simulink model "RTS_15km"  (R2018a)
settings: Solver=ode15s  StartTime=0.0  StopTime=20  FixedStep=0.00001  RelTol=1e-3  AbsTol=1e-6
values from neighbouring files (symbols this model uses):
  ADAMS_cwd = 'C:\Users\gct14001\Documents\Latest DECEMBER Bike Model\Simulation Files'    [Nonlinear_Torque_15km.m]
  ADAMS_exec = ''    [Nonlinear_Torque_15km.m]
  ADAMS_host = 'DESKTOP-F3FKN9V.mdh.se'    [Nonlinear_Torque_15km.m]
  ADAMS_init = ''    [Nonlinear_Torque_15km.m]
  ADAMS_inputs = 'TorqueMotor.var_motor_torque!V_In!FrameDisturbance'    [Nonlinear_Torque_15km.m]
  ADAMS_outputs = 'LeanAng_In!SteerAngle!V_Out!Dist!DriftAngle'    [Nonlinear_Torque_15km.m]
  ADAMS_prefix = 'Nonlinear_Torque_15km'    [Nonlinear_Torque_15km.m]
  ADAMS_static = 'no'    [Nonlinear_Torque_15km.m]
  ADAMS_sysdir = 'C:\PROGRA~1\MSC~1.SOF\ADAMSS~1\2018_1\'    [Nonlinear_Torque_15km.m]
  Cline = v*inv(M)*C1    [DynamicModelParameters.m]
  Kline = inv(M)*(g*K0+v^2*K2)    [DynamicModelParameters.m]
  Mline = inv(M)    [DynamicModelParameters.m]
libraries: simulink_extras x3, simulink x2, dspfdesign x1
settings Model: Creator=FoR  LastModifiedBy=gct14001
settings SolverCC: SolverResetMethod=Robust
settings CodeAppCC: StateflowObjectComments=on

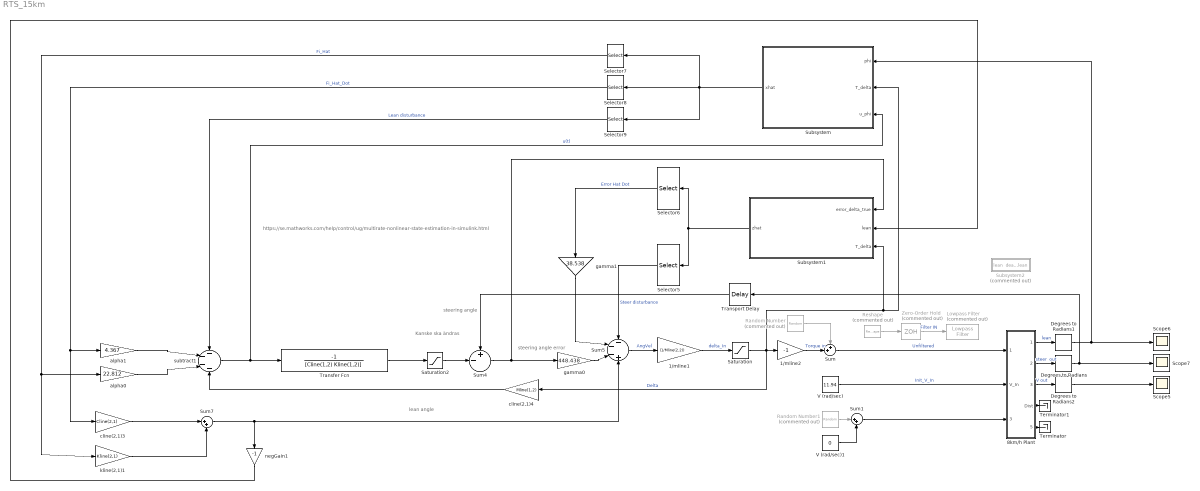
== system RTS_15km ==
  note: steering angle
  note: https://se.mathworks.com/help/control/ug/multirate-nonlinear-state-estimation-in-simulink.html
  note: steering angle error
  note: Kanske ska
      | ändras
  note: lean angle
  1/mline1 : Gain  Gain=(1/Mline(2,2))
  1/mline2 : Gain  Gain=-1
  8km/h Plant : Subsystem
  Degrees to Radians : simulink_extras/Transformations/Degrees to Radians
  Degrees to Radians1 : simulink_extras/Transformations/Degrees to Radians
  Degrees to Radians2 : simulink_extras/Transformations/Degrees to Radians
  Lowpass Filter : dspfdesign/Lowpass Filter  Commented=on  FilterType=FIR  DesignForMinimumOrder=on  FilterOrder=50  PassbandFrequency=15  StopbandFrequency=50  PassbandRipple=0.1  StopbandAttenuation=80  InheritSampleRate=off  SampleRate=44100  SimulateUsing=Interpreted execution  roundingMode=Floor  coeffsDataTypeStr=fixdt(1,16)
  Random Number : RandomNumber  Commented=on  Variance=0.1  SampleTime=0.1
  Random Number1 : RandomNumber  Commented=on  Variance=0.1  SampleTime=0.1
  Reshape : Reshape  Commented=on  OutputDimensionality=Customize  OutputDimensions=1
  Saturation : Saturate  UpperLimit=12  LowerLimit=-12
  Saturation2 : Saturate  UpperLimit=90  LowerLimit=-90
  Scope5 : Scope
  Scope6 : Scope
  Scope7 : Scope
  Selector5 : Selector  InputPortWidth=6  IndexOptions=Index vector (dialog)  Indices=3  OutputSizes=1
  Selector6 : Selector  InputPortWidth=6  IndexOptions=Index vector (dialog)  Indices=2  OutputSizes=1
  Selector7 : Selector  InputPortWidth=3  IndexOptions=Index vector (dialog)  Indices=1  OutputSizes=1
  Selector8 : Selector  InputPortWidth=3  IndexOptions=Index vector (dialog)  Indices=2  OutputSizes=1
  Selector9 : Selector  InputPortWidth=3  IndexOptions=Index vector (dialog)  Indices=3  OutputSizes=1
  Subsystem : Subsystem
  Subsystem1 : Subsystem
  Subsystem2 : Subsystem  Commented=on
  Sum : Sum  Inputs=++|
  Sum1 : Sum  Inputs=|++
  Sum4 : Sum  Inputs=+-|
  Sum5 : Sum  Inputs=---+
  Sum7 : Sum  Inputs=|++
  Terminator : Terminator
  Terminator1 : Terminator
  Transfer Fcn : TransferFcn  Numerator=[-1]  Denominator=[Cline(1,2) Kline(1,2)]
  Transport Delay : TransportDelay  DelayTime=0.005
  V (rad/sec) : Constant  Value=11.94
  V (rad/sec)1 : Constant  Value=0
  Zero-Order Hold : ZeroOrderHold  Commented=on  SampleTime=-1
  alpha0 : Gain  Gain=22.812
  alpha1 : Gain  Gain=4.367
  cline(2,1)3 : Gain  Gain=Cline(2,1)
  cline(2,1)4 : Gain  Gain=Mline(1,2)
  gamma0 : Gain  Gain=448.438
  "gamma1 " : Gain  Gain=38.538
  kline(2,1)1 : Gain  Gain=Kline(2,1)
  negGain1 : Gain  Gain=-1
  subtract1 : Sum  Inputs=----
  wires:
  Saturation/1 -> 1/mline2/1, cline(2,1)4/1, Subsystem1/3(T_delta), Subsystem/2(T_delta)  "Delta"
  Subsystem1/1(zhat) -> Selector5/1, Selector6/1
  Selector7/1 -> kline(2,1)1/1, alpha0/1  "Fi_Hat"
  cline(2,1)3/1 -> Sum7/1
  Selector9/1 -> subtract1/1  "Lean disturbance"
  cline(2,1)4/1 -> subtract1/4
  Selector5/1 -> Sum5/1  "Steer disturbance"
  Sum7/1 -> negGain1/1, Sum5/4
  Sum5/1 -> 1/mline1/1  "AngVel"
  alpha0/1 -> subtract1/3
  alpha1/1 -> subtract1/2
  gamma0/1 -> Sum5/3
  kline(2,1)1/1 -> Sum7/2
  subtract1/1 -> Transfer Fcn/1, Subsystem/3(u_phi)  "u(t)"
  1/mline1/1 -> Saturation/1  "delta_In"
  Selector8/1 -> cline(2,1)3/1, alpha1/1  "Fi_Hat_Dot"
  8km/h Plant/3("V_Out     ") -> Degrees to Radians2/1  "V out"
  "gamma1 "/1 -> Sum5/2
  Sum4/1 -> Subsystem1/1(error_delta_true), gamma0/1
  Selector6/1 -> "gamma1 "/1  "Error Hat Dot"
  Saturation2/1 -> Sum4/2
  negGain1/1 -> Subsystem1/2(lean)
  Subsystem/1(xhat) -> Selector9/1, Selector8/1, Selector7/1
  V (rad/sec)/1 -> 8km/h Plant/2("V_In                        ")  "Init_V_In"
  8km/h Plant/4("Dist      ") -> Terminator1/1
  8km/h Plant/5(DriftAngle) -> Terminator/1
  8km/h Plant/2(SteerAngle) -> Degrees to Radians/1  "steer  out"
  Transfer Fcn/1 -> Saturation2/1
  Degrees to Radians/1 -> Scope7/1, Transport Delay/1
  Transport Delay/1 -> Sum4/1
  Degrees to Radians1/1 -> Subsystem/1(phi), Scope6/1
  1/mline2/1 -> Sum/2  "Torque in"
  Random Number/1 -> Sum/1
  8km/h Plant/1(LeanAng_In) -> Degrees to Radians1/1  "lean"
  V (rad/sec)1/1 -> Sum1/2
  Degrees to Radians2/1 -> Scope5/1
  Random Number1/1 -> Sum1/1
  Sum1/1 -> 8km/h Plant/3("FrameDisturbance            ")
  Sum/1 -> 8km/h Plant/1(TorqueMotor.var_motor_torque)  "Unfiltered"
  Reshape/1 -> Zero-Order Hold/1
  Zero-Order Hold/1 -> Lowpass Filter/1  "Filter IN"

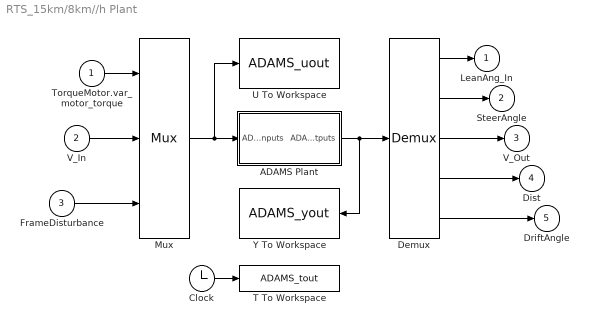
== system RTS_15km/8km//h Plant ==
  TorqueMotor.var_motor_torque : Inport
  "V_In                        " : Inport  Port=2
  "FrameDisturbance            " : Inport  Port=3
  ADAMS Plant : Subsystem  LoadFcn=|  InitFcn=clear mex  mask(Adams Plant){exevie=ADAMS_sysdir, nam_in=ADAMS_inputs, namout=ADAMS_outputs, nampre=ADAMS_prefix, outfil=ADAMS_prefix, exesol=ADAMS_exec, stat=ADAMS_static, inicmd=[ADAMS_init], exetyp=C++, comtyp=PIPE(DDE), workdir=ADAMS_cwd, ada_host=ADAMS_host, modani=batch, modsim=discrete, dft=no, simulink_lead_cosim=yes, pin_interp_order=0, pout_extrap_order=0, pin_extrap_order=0, pout_interp_order=0, dt_out=0.005, o_rate=1, more=off}
      | %check based on dialog box setting for when setting by popup menu                                             
      | if exist('ADAMS_solver_type')                                                                                 
      |   if strcmp(ADAMS_solver_type,'C++')                                                                          
      |     set_param(gcb,'exetyp','C++');                                                                            
      |   else                                                                                                        
      |     set_param(gcb,'exetyp','Fortran');                                                                        
      |   end                                                                                                         
      | else                                                                                                          
      |   set_param(gcb,'exetyp','C++');                                                                              
      | end                                                                                                           
      | %set the mode if using acar_solver                                                                            
      | %REQUIRED HERE BECAUSE BELOW CAUSES MDLTERMINATE TO BE CALLED 2 TIMES IN MIDDLE OF SIMULATION WHEN SET IN MASK
      |                                                                                                               
      | %enable the direct feedthrough, sim mode, anim mode parameters by default                                     
      |                                                                                                               
      | if exist('set_some_params_states')                                                                            
      |                                                                                                               
      |   set_some_params_states({'dft','modsim','modani'},{'on','on','on'},'MaskEnables',gcb)                        
      |   %turn on direct feedthrough option                                                                          
      |   set_some_params_states({'dft'},{'on'},'MaskVisibilities',gcb)                                               
      |                                                                                                               
      |  end                                                                                                          
      |                                                                                                               
      |                                                                                                               
      | if exist('ADAMS_exec')                                                                                        
      |   if and(strcmp(get_param(gcb,'exesol'),'ADAMS_exec'),strcmp(ADAMS_exec,'acar_solver'))                       
      |     %set the sim mode to discrete -- only supported mode                                                      
      |     set_param(gcb,'modsim','discrete')                                                                        
      |      %turn off direct feedthrough option                                                                      
      |      set_some_params_states({'dft'},{'off'},'MaskVisibilities',gcb)                                           
      |     %set the animation mode to batch -- only supported mode                                                   
      |     set_param(gcb,'modani','batch')                                                                           
      |     %disable the direct feedthrough, sim mode, anim mode parameters                                           
      |     set_some_params_states({'modsim','modani'},{'off','off'},'MaskEnables',gcb)                               
      |   end                                                                                                         
      | end
      mask prompts: exevie "Adams install directory"; nam_in "Adams View input names"; namout "Adams View output names"; nampre "Adams model file prefix"; outfil "Output files prefix (opt.: if blank - no output)"; exesol "User executable (opt.: if blank - use standard)"; stat "Initial static simulation flag"; inicmd "Initialization commands"; exetyp "Adams Solver type"; comtyp "Interprocess option"; workdir "Adams working directory"; ada_host "Adams host"; modani "Animation mode"; modsim "Simulation mode"; dft "Direct feedthrough"; simulink_lead_cosim "Discrete Computational Order - Simulink Leads Adams"; pin_interp_order "Plant input interpolation order"; pout_extrap_order "Plant output extrapolation order"; pin_extrap_order "Plant input extrapolation order"; pout_interp_order "Plant output interpolation order"; dt_out "Communication interval"; o_rate "Number of communications per output step"; more "More parameters"
      mask help: Simulate any Adams plant model either in Adams Solver form (.adm file) or in Adams View form (.cmd file)
      settings: OpenFcn=|
      | open_system(gcb,'mask')
      | if not(exist('set_some_params_states'))
      | 
      | warning('The script "set_some_params_states.m" cannot be found in the MATLAB PATH.  Cannot update the ADAMS Plant S-Function parameters.')
      | 
      | warning('Recommended action(optional):  run the Adams Controls .m file first to help choose the correct settings in the Adams S-Function block.')
      | 
      | end
      mask Help:
      | <html>
      | This S-Function represents the non-linear Adams Plant with the inputs sent to the Adams model <br>
      |  and the outputs generated by the Adams model.  See the Adams Controls documentation for more <br>
      | information.  This plant uses the following variables:<br>
      | <br>
      | <b>ADAMS_sysdir  :</b> Adams installation directory<br>
      | <b>ADAMS_inputs  :</b> Input variables View names vector<br>
      | <b>ADAMS_outputs :</b> Outputs variables View names vector<br>
      | <b>ADAMS_prefix  : </b>ADAMS model files prefix (.adm, .cmd); also doubles as output files prefix<br>
      | <b>ADAMS_exec :</b> Adams Solver user library or keyword (e.g., acar_solver)<br>
      | <b>ADAMS_static :</b> yes|no - initial static before Co-simulation(discrete)/Function Evaluation(continuous)<br>
      | <b>ADAMS_init :</b>Initialization commands (i.e., Adams View or Solver commands, depending on setting for Animation mode)<br>
      | <b>ADAMS_cwd : </b> Current working directory (for TCP/IP)<br>
      | <b>ADAMS_host : </b>Name of Adams server host (for TCP/IP)<br>
      | <b>ADAMS_mode :</b> Linear or non-linear (i.e., co-sim, function eval)<br>
      | <b>ADAMS_solver_type :</b>Fortran or C++ (used to set popup menu when first loaded) <br>
      | 
      | 
      | <br>
      | The following settings can be chosen:<br>
      | <br>
      | <b>Adams Solver type:</b>  Fortran or C++ (will also set ADAMS_solver_type)<br>
      | <b>Interprocess option:</b> Pipe(DDE) or TCP/IP; TCP/IP can allow different machines run Adams and MATLAB<br>
      | <b>Animation mode:</b> batch (Solver, uses .adm) or interactive (View, uses .cmd)<br>
      | <b>Simulation mode:</b> discrete (Co-simulation) or continuous (Function Evaluation)<br>
      | <b>Discrete Computational Order - Simulink Lead Adams:</b> for discrete mode, chooses if Simulink leads the integration (yes) or lags (no);<br> if set to "no", can remove algebraic loop<br>
      | <b>Plant input interpolation order:</b> 0 = zero-order hold; 1 = linear (discrete mode only, where Simulink leads)<br>
      | <b>Plant output extrapolation order:</b> 0 = zero-order hold;1 = linear(discrete mode only, where Simulink leads)<br>
      | <b>Plant input extrapolation order:</b> 0 = zero-order hold; 1 = linear (discrete mode only, where Adams leads)<br>
      | <b>Plant output interpolation order:</b> 0 = zero-order hold;1 = linear(discrete mode only, where Adams leads)<br>
      | <b>Direct feedthrough:</b> yes|no - yes = Input directly effect output(continuous mode-only)<br>
      | <b>Communication interval:</b> Time step at which Co-simulation exchange information (e.g.,0.005); also controls <br>output for continuous mode (Function Evaluation)<br>
      | <b>Number of communications per output step: </b>Sets Adams output rate (.res, .req, .gra) integer value (default: 1)<br>
      | </html>
      mask Callback exesol:
      | if exist('set_some_params_states')
      | %enable the direct feedthrough, sim mode, anim mode parameters
      | set_some_params_states({'dft','modsim','modani'},{'on','on','on'},'MaskEnables',gcb)
      | %turn on direct feedthrough option
      | set_some_params_states({'dft'},{'on'},'MaskVisibilities',gcb)
      | end
      | 
      | if exist('ADAMS_exec')
      |   if and(strcmp(get_param(gcb,'exesol'),'ADAMS_exec'),strcmp(ADAMS_exec,'acar_solver'))
      |     %set the sim mode to discrete -- only supported mode
      |     %REMOVED:  BELOW CAUSES MDLTERMINATE TO BE CALLED 2 TIMES IN MIDDLE OF SIMULATION
      |     %Now in LoadFcn callback
      |     %set_param(gcb,'modsim','discrete')
      |      %turn off direct feedthrough option
      |     set_some_params_states({'dft'},{'off'},'MaskVisibilities',gcb)
      |     %set the animation mode to batch -- only supported mode
      |     %REMOVED:  BELOW CAUSES MDLTERMINATE TO BE CALLED 2 TIMES IN MIDDLE OF SIMULATION
      |     %Now in LoadFcn callback
      |     %set_param(gcb,'modani','batch')
      |     %disable the direct feedthrough, sim mode, anim mode parameters
      |     set_some_params_states({'modsim','modani'},{'off','off'},'MaskEnables',gcb)
      |   end
      | end
      mask TypeOptions exetyp: Fortran | C++
      mask Callback exetyp:
      | if strcmp(get_param(gcb,'exetyp'),'C++')
      |     ADAMS_solver_type='C++';
      | else
      |     ADAMS_solver_type='Fortran';
      | end
      mask TypeOptions comtyp: PIPE(DDE) | TCP/IP
      mask Callback comtyp:
      | if exist('set_some_params_states')
      | if strcmp(get_param(gcb,'comtyp'),'PIPE(DDE)')
      |     %turn off cwd, host options
      |     set_some_params_states({'ada_host','workdir'},{'off','off'},'MaskVisibilities',gcb)
      | else%if strcmp(get_param(gcb,'modsim'),'TCP/IP')
      |     %turn on cwd, host options
      |     set_some_params_states({'ada_host','workdir'},{'on','on'},'MaskVisibilities',gcb)
      | end
      | end
      mask TypeOptions modani: batch | interactive
      mask TypeOptions modsim: discrete | continuous
      mask Callback modsim:
      | if exist('set_some_params_states')
      | if strcmp(get_param(gcb,'modsim'),'discrete')
      |      %turn off direct feedthrough option
      |     set_some_params_states({'dft'},{'off'},'MaskVisibilities',gcb)
      |     %turn on discrete co-sim type if want to see more
      |     if strcmp(get_param(gcb,'more'),'on')
      |         set_some_params_states({'simulink_lead_cosim'},{'on'},'MaskVisibilities',gcb)
      |     end
      |     if strcmp(get_param(gcb,'simulink_lead_cosim'),'yes')
      |         %turn on interpolation/extrapolation options
      |         set_some_params_states({'pin_interp_order','pout_extrap_order',},{'on','on'},'MaskVisibilities',gcb)
      |     else
      |         set_some_params_states({'pin_extrap_order','pout_interp_order'},{'on','on'},'MaskVisibilities',gcb)
      |     end
      | else%if strcmp(get_param(gcb,'modsim'),'continuous')
      |      %turn off direct feedthrough option
      |     set_some_params_states({'dft'},{'on'},'MaskVisibilities',gcb)
      |     %turn off interpolation/extrapolation options
      |     set_some_params_states({'pin_interp_order','pout_extrap_order','pin_extrap_order','pout_interp_order','simulink_lead_cosim'},{'off','off','off','off','off'},'MaskVisibilities',gcb)
      | end
      | end
      mask TypeOptions dft: no | yes
      mask TypeOptions simulink_lead_cosim: yes | no
      mask Callback simulink_lead_cosim:
      | if exist('set_some_params_states')
      | if (strcmp(get_param(gcb,'simulink_lead_cosim'),'yes') && strcmp(get_param(gcb,'modsim'),'discrete'))
      |      %turn off unused interpolate/extrapolate options
      |     set_some_params_states({'pin_extrap_order','pout_interp_order'},{'off','off'},'MaskVisibilities',gcb)
      |     %turn on used interpolate/extrapolate options
      |     set_some_params_states({'pin_interp_order','pout_extrap_order'},{'on','on'},'MaskVisibilities',gcb)
      | elseif (strcmp(get_param(gcb,'simulink_lead_cosim'),'no') && strcmp(get_param(gcb,'modsim'),'discrete'))
      |     %turn on used interpolate/extrapolate options
      |     set_some_params_states({'pin_extrap_order','pout_interp_order'},{'on','on'},'MaskVisibilities',gcb)
      |      %turn off unused interpolate/extrapolate options
      |     set_some_params_states({'pin_interp_order','pout_extrap_order'},{'off','off'},'MaskVisibilities',gcb)
      | end
      | end
      mask TypeOptions pin_interp_order: 0 | 1
      mask TypeOptions pout_extrap_order: 0 | 1
      mask TypeOptions pin_extrap_order: 0 | 1
      mask TypeOptions pout_interp_order: 0 | 1
      mask Callback more:
      | if exist('set_some_params_states')
      | if (strcmp(get_param(gcb,'more'),'on'))
      |      %turn on infrequently used options
      |     set_some_params_states({'exevie','nam_in','namout','exesol','stat','inicmd'},{'on','on','on','on','on','on'},'MaskVisibilities',gcb)
      |     if strcmp(get_param(gcb,'modsim'),'discrete')
      |         set_some_params_states({'simulink_lead_cosim'},{'on'},'MaskVisibilities',gcb)
      |     end
      | elseif (strcmp(get_param(gcb,'more'),'off'))
      |     %turn off infrequently used options
      |     set_some_params_states({'exevie','nam_in','namout','exesol','stat','inicmd'},{'off','off','off','off','off','off'},'MaskVisibilities',gcb)
      |     if strcmp(get_param(gcb,'modsim'),'discrete')
      |         set_some_params_states({'simulink_lead_cosim'},{'off'},'MaskVisibilities',gcb)
      |     end
      | end
      | end
      mask Display: disp( 'MSC Software' )
  Clock : Clock
  Demux : Demux  Outputs=5
  Mux : Mux  Inputs=3
  T To Workspace : ToWorkspace  VariableName=ADAMS_tout
      settings: MaxDataPoints=100000
  U To Workspace : ToWorkspace  VariableName=ADAMS_uout
      settings: MaxDataPoints=100000
  Y To Workspace : ToWorkspace  VariableName=ADAMS_yout
      settings: MaxDataPoints=100000
  LeanAng_In : Outport
  SteerAngle : Outport  Port=2
  "V_Out     " : Outport  Port=3
  "Dist      " : Outport  Port=4
  DriftAngle : Outport  Port=5
  wires:
  "FrameDisturbance            "/1 -> Mux/3
  "V_In                        "/1 -> Mux/2
  TorqueMotor.var_motor_torque/1 -> Mux/1
  Demux/5 -> DriftAngle/1
  Demux/4 -> "Dist      "/1
  Demux/3 -> "V_Out     "/1
  Demux/2 -> SteerAngle/1
  Demux/1 -> LeanAng_In/1
  ADAMS Plant/1(ADAMS outputs) -> Y To Workspace/1, Demux/1
  Mux/1 -> U To Workspace/1, ADAMS Plant/1(ADAMS inputs)
  Clock/1 -> T To Workspace/1

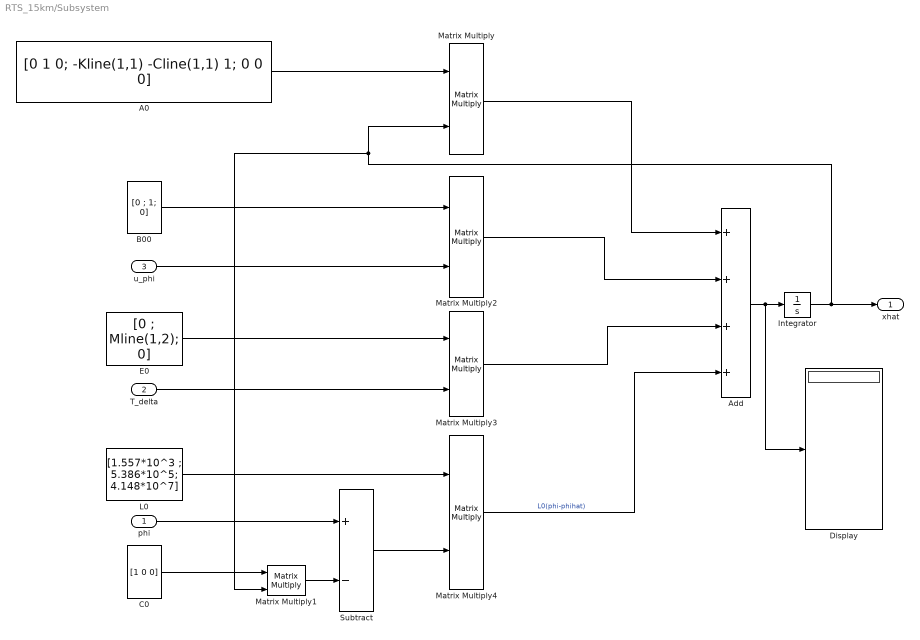
== system RTS_15km/Subsystem ==
  phi : Inport
  T_delta : Inport  Port=2
  u_phi : Inport  Port=3
  A0 : Constant  Value=[0 1 0; -Kline(1,1) -Cline(1,1) 1; 0 0 0]
  Add : Sum  Inputs=++++
  B00 : Constant  Value=[0 ; 1; 0]  VectorParams1D=off
  C0 : Constant  Value=[1 0 0]  VectorParams1D=off
  Display : Display
  "E0 " : Constant  Value=[0 ; Mline(1,2); 0]  VectorParams1D=off
  Integrator : Integrator
  L0 : Constant  Value=[1.557*10^3 ; 5.386*10^5; 4.148*10^7]  VectorParams1D=off
  Matrix Multiply{,1..4} (5 alike) : Product  Multiplication=Matrix(*)
  Subtract : Sum  Inputs=+-
  xhat : Outport
  wires:
  A0/1 -> Matrix Multiply/1
  B00/1 -> Matrix Multiply2/1
  u_phi/1 -> Matrix Multiply2/2
  "E0 "/1 -> Matrix Multiply3/1
  T_delta/1 -> Matrix Multiply3/2
  C0/1 -> Matrix Multiply1/1
  Matrix Multiply1/1 -> Subtract/2
  phi/1 -> Subtract/1
  Subtract/1 -> Matrix Multiply4/2
  L0/1 -> Matrix Multiply4/1
  Matrix Multiply/1 -> Add/1
  Matrix Multiply2/1 -> Add/2
  Matrix Multiply3/1 -> Add/3
  Matrix Multiply4/1 -> Add/4  "L0(phi-phihat)"
  Add/1 -> Display/1, Integrator/1
  Integrator/1 -> xhat/1, Matrix Multiply1/2, Matrix Multiply/2

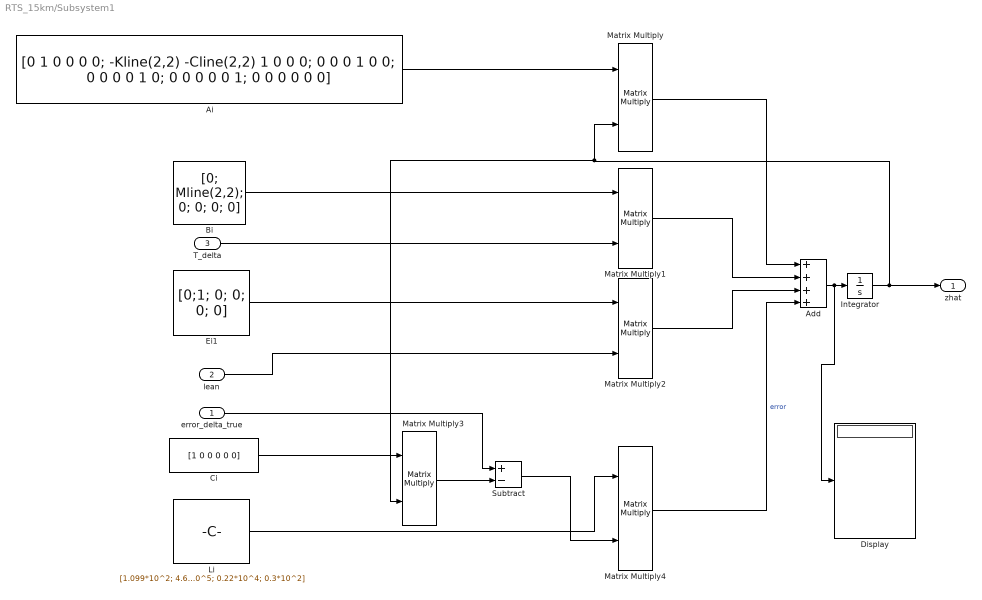
== system RTS_15km/Subsystem1 ==
  error_delta_true : Inport
  lean : Inport  Port=2
  T_delta : Inport  Port=3
  Add : Sum  Inputs=++++
  Ai : Constant  Value=[0 1 0 0 0 0; -Kline(2,2) -Cline(2,2) 1 0 0 0; 0 0 0 1 0 0; 0 0 0 0 1 0; 0 0 0 0 0 1; 0 0 0 0 0 0]
  Bi : Constant  Value=[0; Mline(2,2); 0; 0; 0; 0]  VectorParams1D=off
  Ci : Constant  Value=[1 0 0 0 0 0]  VectorParams1D=off
  Display : Display
  Ei1 : Constant  Value=[0;1; 0; 0; 0; 0]  VectorParams1D=off
  Integrator : Integrator
  Li : Constant  Value=[1.099*10^2; 4.693*10^3; 1.094*10^5; 0.22*10^5; 0.22*10^4; 0.3*10^2]  VectorParams1D=off
  Matrix Multiply{,1..4} (5 alike) : Product  Multiplication=Matrix(*)
  Subtract : Sum  Inputs=+-
  zhat : Outport
  wires:
  T_delta/1 -> Matrix Multiply1/2
  Bi/1 -> Matrix Multiply1/1
  Ai/1 -> Matrix Multiply/1
  Ei1/1 -> Matrix Multiply2/1
  lean/1 -> Matrix Multiply2/2
  Matrix Multiply/1 -> Add/1
  Matrix Multiply1/1 -> Add/2
  Matrix Multiply2/1 -> Add/3
  Ci/1 -> Matrix Multiply3/1
  error_delta_true/1 -> Subtract/1
  Matrix Multiply3/1 -> Subtract/2
  Matrix Multiply4/1 -> Add/4  "error"
  Subtract/1 -> Matrix Multiply4/2
  Li/1 -> Matrix Multiply4/1
  Add/1 -> Display/1, Integrator/1
  Integrator/1 -> Matrix Multiply3/2, Matrix Multiply/2, zhat/1

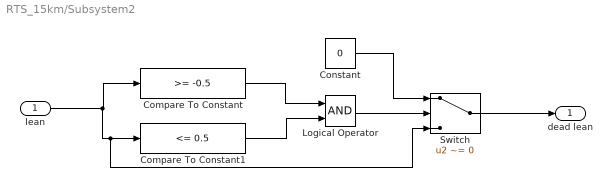
== system RTS_15km/Subsystem2 ==
  lean : Inport
  Compare To Constant : simulink/Logic and Bit Operations/Compare To Constant  relop=>=  const=-0.5  OutDataTypeStr=boolean
  Compare To Constant1 : simulink/Logic and Bit Operations/Compare To Constant  relop=<=  const=0.5  OutDataTypeStr=boolean
  Constant : Constant  Value=0
  Logical Operator : Logic  AllPortsSameDT=off  OutDataTypeStr=boolean
  Switch : Switch  Criteria=u2 ~= 0
  dead lean : Outport
  wires:
  Switch/1 -> dead lean/1
  Compare To Constant1/1 -> Logical Operator/2
  lean/1 -> Switch/3, Compare To Constant1/1, Compare To Constant/1
  Logical Operator/1 -> Switch/2
  Compare To Constant/1 -> Logical Operator/1
  Constant/1 -> Switch/1

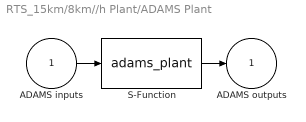
== system RTS_15km/8km//h Plant/ADAMS Plant ==
  ADAMS inputs : Inport
  S-Function : S-Function  StopFcn=clear mex  FunctionName=adams_plant  Parameters=exevie,exesol,stat,outfil,nampre,o_rate,nam_in,namout,dft,modsim,modani,dt_out,inicmd,exetyp,comtyp,ada_host, workdir,pin_interp_order,pout_extrap_order,pin_extrap_order,pout_interp_order,simulink_lead_cosim  SFunctionDeploymentMode=off  EnableBusSupport=off
  ADAMS outputs : Outport  InitialOutput=0
  wires:
  S-Function/1 -> ADAMS outputs/1
  ADAMS inputs/1 -> S-Function/1
